simulink model "FederMasseGedaempft"  (Simulink 7.1)
settings: Solver=ode45  StartTime=0.0  StopTime=1.0  RelTol=1e-3
settings Model: Creator=Meisel  LastModifiedBy=Meisel

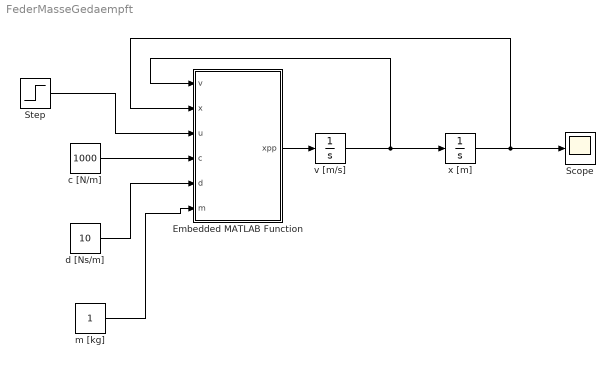
== system FederMasseGedaempft ==
  Embedded MATLAB Function : Stateflow chart
  Scope : Scope
      settings: TimeRange=1  YMin=0  YMax=0.2
  Step : Step  Time=0  After=0.1  SampleTime=0
  c [N/m] : Constant  Value=1000  OutDataType=sfix(16)  OutScaling=2^0
  d [Ns/m] : Constant  Value=10  OutDataType=sfix(16)  OutScaling=2^0
  m [kg] : Constant  OutDataType=sfix(16)  OutScaling=2^0
  v [m/s] : Integrator
  x [m] : Integrator
  wires:
  v [m/s]/1 -> x [m]/1, Embedded MATLAB Function/1(v)
  Embedded MATLAB Function/1(xpp) -> v [m/s]/1
  c [N/m]/1 -> Embedded MATLAB Function/4(c)
  d [Ns/m]/1 -> Embedded MATLAB Function/5(d)
  m [kg]/1 -> Embedded MATLAB Function/6(m)
  x [m]/1 -> Embedded MATLAB Function/2(x), Scope/1
  Step/1 -> Embedded MATLAB Function/3(u)

== matlab function Embedded MATLAB Function ==
  data: v input double; x input double; u input double; xpp output double; c input double; d input double; m input double
function xpp = fcn(v,x,u,c,d,m)
% This block supports the Embedded MATLAB subset.
% See the help menu for details. 

xpp = 1/m*((u-x)*c-v*d);
